simulink model "Ebike"  (R2024b)
settings: Solver=VariableStepAuto  StartTime=0.0  StopTime=20.0  RelTol=1e-3
settings Model: Creator=s.maatoug  LastModifiedBy=s.maatoug

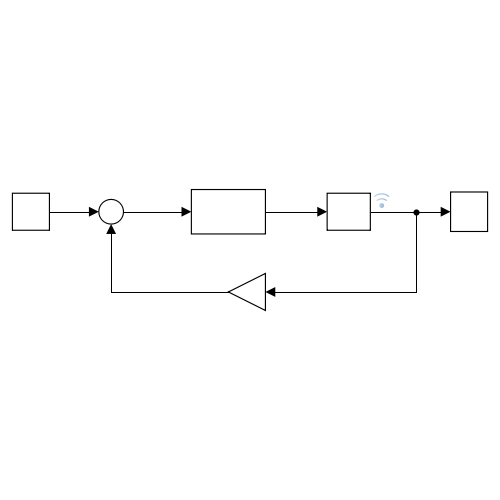
[thumbnail: Simulink's stored preview of the top-level diagram]
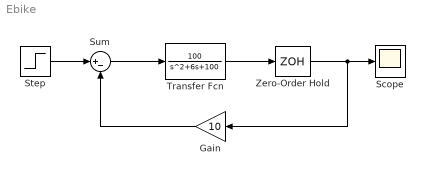
== system Ebike ==
  Gain : Gain  Gain=10
  Scope : Scope
  Step : Step  SampleTime=0
  Sum : Sum  Inputs=|+-
  Transfer Fcn : TransferFcn  Numerator=[100]  Denominator=[1 6 100]
  Zero-Order Hold : ZeroOrderHold  SampleTime=0.01
  wires:
  Step/1 -> Sum/1
  Sum/1 -> Transfer Fcn/1
  Transfer Fcn/1 -> Zero-Order Hold/1
  Gain/1 -> Sum/2
  Zero-Order Hold/1 -> Gain/1, Scope/1
